simulink model "Ques7Ex3_AkankshaMurali"  (R2023b)
settings: Solver=VariableStepAuto  StartTime=0.0  StopTime=10.0  RelTol=1e-3
settings Model: Creator=akank  LastModifiedBy=akank

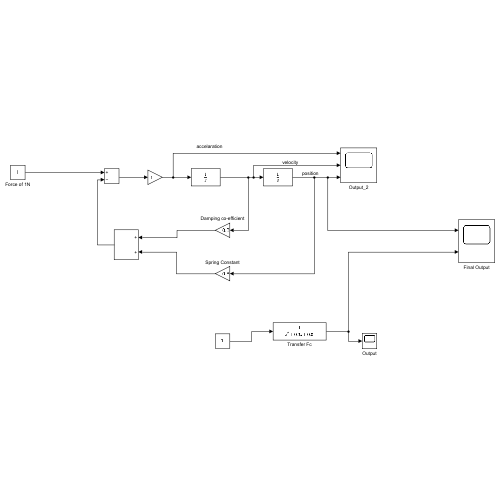
[thumbnail: Simulink's stored preview of the top-level diagram]
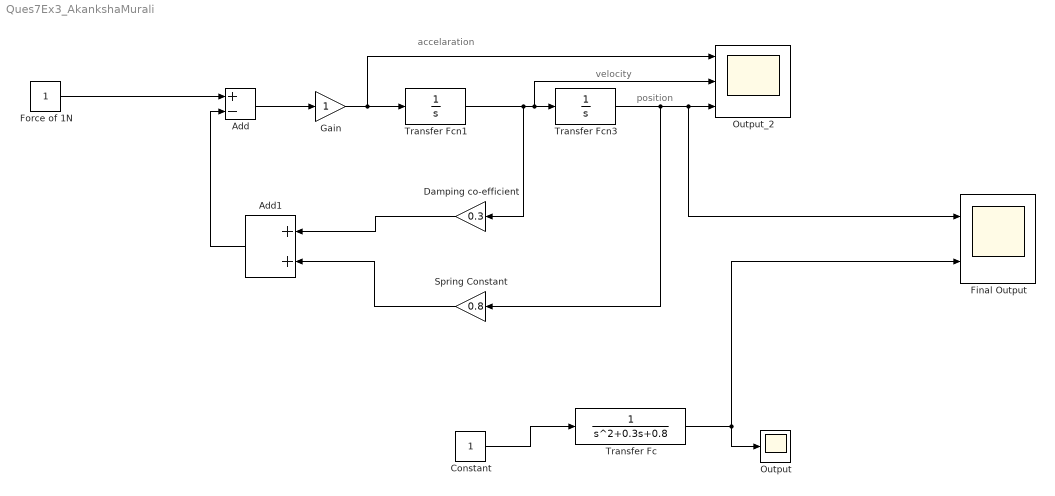
== system Ques7Ex3_AkankshaMurali ==
  note: position
  note: velocity
  note: accelaration
  Add : Sum  Inputs=+-
  Add1 : Sum
  Constant : Constant
  Damping co-efficient : Gain  Gain=0.3
  Final Output : Scope  NumInputPorts=2
  Force of 1N : Constant
  Gain : Gain
  Output : Scope
  Output_2 : Scope  NumInputPorts=3
  Spring Constant : Gain  Gain=0.8
  Transfer Fc : TransferFcn  Denominator=[1 0.3 0.8]
  Transfer Fcn1 : TransferFcn  Denominator=[1 0]
  Transfer Fcn3 : TransferFcn  Denominator=[1 0]
  wires:
  Add/1 -> Gain/1
  Gain/1 -> Output_2/1, Transfer Fcn1/1
  Force of 1N/1 -> Add/1
  Add1/1 -> Add/2
  Spring Constant/1 -> Add1/2
  Damping co-efficient/1 -> Add1/1
  Constant/1 -> Transfer Fc/1
  Transfer Fcn1/1 -> Damping co-efficient/1, Output_2/2, Transfer Fcn3/1
  Transfer Fcn3/1 -> Final Output/1, Output_2/3, Spring Constant/1
  Transfer Fc/1 -> Output/1, Final Output/2
